simulink model "BLT_HPF"  (R2020a)
settings: Solver=VariableStepAuto  StartTime=0.0  StopTime=10  RelTol=1e-3
settings Model: Creator=I3  LastModifiedBy=I3

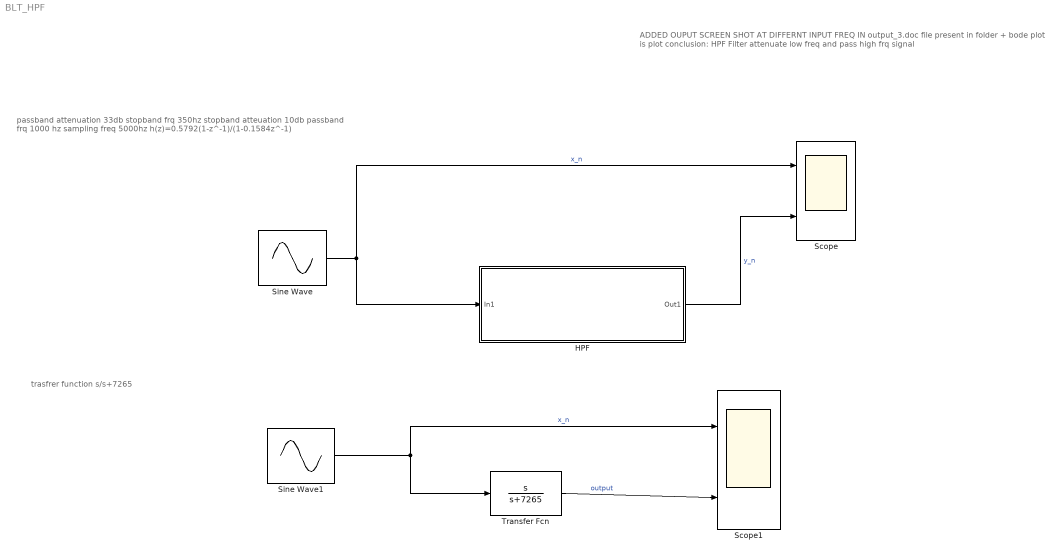
== system BLT_HPF ==
  note: ADDED OUPUT SCREEN SHOT AT DIFFERNT INPUT FREQ IN output_3.doc file present in folder + bode plot is plot
      | conclusion:
      | HPF Filter attenuate low freq and pass high frq signal
  note: trasfrer function
      | s/s+7265
  note: passband attenuation 33db stopband frq 350hz
      | stopband atteuation 10db passband frq 1000 hz
      | sampling freq 5000hz
      |
      | h(z)=0.5792(1-z^-1)/(1-0.1584z^-1)
  HPF : Subsystem
  Scope : Scope  NumInputPorts=2
  Scope1 : Scope  NumInputPorts=2
  Sine Wave : Sin  Frequency=7500*6.28  SampleTime=2*10^-4
  Sine Wave1 : Sin  Frequency=7500*6.28  SampleTime=0
  Transfer Fcn : TransferFcn  Numerator=[1 0]  Denominator=[1 7265]
  wires:
  Transfer Fcn/1 -> Scope1/2  "output"
  HPF/1(Out1) -> Scope/2  "y_n"
  Sine Wave/1 -> HPF/1(In1), Scope/1  "x_n"
  Sine Wave1/1 -> Transfer Fcn/1, Scope1/1  "x_n"

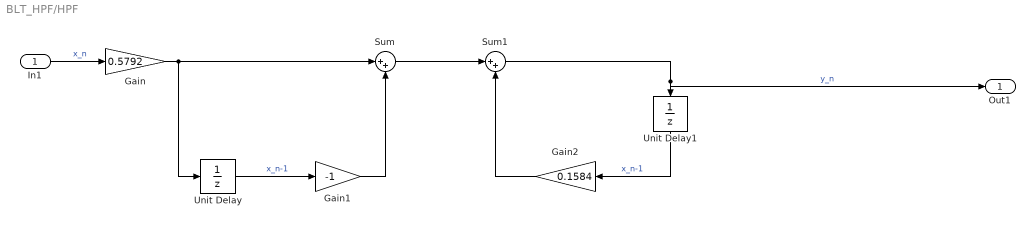
== system BLT_HPF/HPF ==
  In1 : Inport
  Gain : Gain  Gain=0.5792
  Gain1 : Gain  Gain=-1
  Gain2 : Gain  Gain=0.1584
  Sum : Sum  Inputs=|++
  Sum1 : Sum  Inputs=|++
  Unit Delay : UnitDelay  SampleTime=-1  HasFrameUpgradeWarning=on
  Unit Delay1 : UnitDelay  SampleTime=-1  HasFrameUpgradeWarning=on
  Out1 : Outport
  wires:
  In1/1 -> Gain/1  "x_n"
  Sum1/1 -> Out1/1, Unit Delay1/1  "y_n"
  Unit Delay1/1 -> Gain2/1  "x_n-1"
  Unit Delay/1 -> Gain1/1  "x_n-1"
  Gain1/1 -> Sum/2
  Sum/1 -> Sum1/1
  Gain/1 -> Unit Delay/1, Sum/1
  Gain2/1 -> Sum1/2
